simulink model "sampleModel140"  (R2021b)
settings: Solver=VariableStepAuto  StartTime=0.0  StopTime=10.0  RelTol=1e-3
undefined symbols (not defined in the file or in its folder): DiscIntNeverNeededParam, Newton, Raphson
libraries: simulink x11, slpidlib x1
settings Model: Creator=user  LastModifiedBy=user

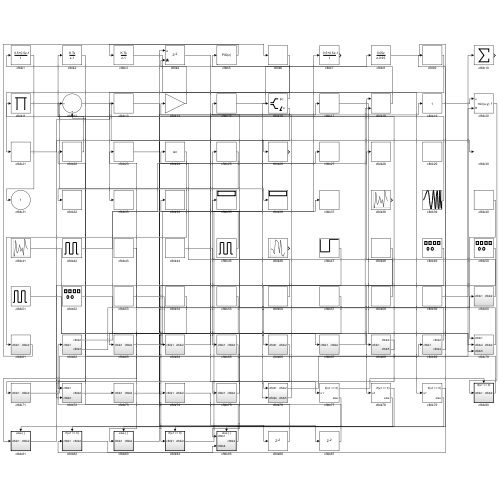
[thumbnail: Simulink's stored preview of the top-level diagram]
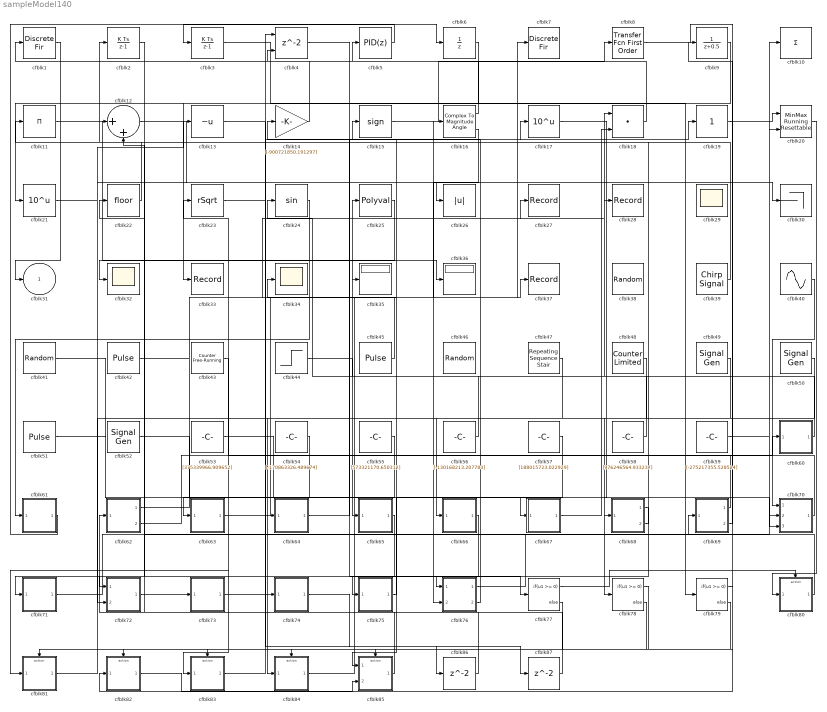
== system sampleModel140 ==
  cfblk1 : DiscreteFir  SampleTime=1
  cfblk10 : Sum  Inputs=+
  cfblk11 : Product  Inputs=*
  cfblk12 : Sum  Inputs=|++
  cfblk13 : UnaryMinus
  cfblk14 : Gain  Gain=[-900721850.191297]
  cfblk15 : Signum
  cfblk16 : ComplexToMagnitudeAngle
  cfblk17 : Math  Operator=10^u  SaturateOnIntegerOverflow=on
  cfblk18 : DotProduct  InputSameDT=on  OutDataTypeStr=Inherit: Inherit via internal rule
  cfblk19 : simulink/Math Operations/Slider Gain  gain=1  low=0  high=2
  cfblk2 : DiscreteIntegrator  ICPrevOutput=DiscIntNeverNeededParam  ICPrevScaledInput=DiscIntNeverNeededParam
  cfblk20 : simulink/Math Operations/MinMax Running Resettable  Function=min  vinit=0.0
  cfblk21 : Math  Operator=10^u  SaturateOnIntegerOverflow=on
  cfblk22 : Rounding
  cfblk23 : Sqrt  Operator=rSqrt  AlgorithmType=Newton-Raphson  SaturateOnIntegerOverflow=on
  cfblk24 : Trigonometry
  cfblk25 : Polyval  Coefs=[ +2.081618890e-019, -1.441693666e-014, +4.719686976e-010, -8.536869453e-006, +1.621573104e-001, -8.087801117e+001 ]
  cfblk26 : Abs
  cfblk27 : Record  FileSettingsInternal="{\"entries\":[{\"content\":{\"excelSettings\":{\"content\":{},\"type\":\"Streamout.ExcelSettings\"}},\"type\":\"Streamout.FileSettingStorage\",\"uuid\":\"f7dc172e-85bf-4364-b29a-430d7ad068c6\"}],\"packageUris\":[\"http://schema.mathworks.com/mf0/streamout_blocks/R2020a\"],\"version\":\"1.0\"}"  SignalsInternal="{\"entries\":[{\"content\":{\"signals\":[{\"content\":{\"blockPath\":[\"sampleModel140/cfblk27\"],\"channel\":[],\"dimensions\":[1],\"domain\":\"sampleModel140/cfblk27\",\"lineColor\":\"#fe330a\",\"plots\":[1],\"port\":1,\"sid\":[\"\"],\"signalID\":4999,\"signalName\":\"cfblk62:1\"},\"type\":\"RecordBlkView.Signal\",\"uuid\":\"44b31170-ca03-488e-82e6-39e71cb301d7\"}]},\"type\":\"RecordBlkView.InputSignals\",\"uuid\":\"1dfdc35e-76fa-4b09-975a-dfabfb6ba794\"}],\"packageUris\":[\"http://schema.mathworks.com/mf0/streamout_blocks/R2020a\"],\"version\":\"1.0\"}"  VisualizationBindings="{\"sparklinesplugin\":{\"info\":[{\"bindingParametersList\":[],\"subplotID\":1}]}}"
  cfblk28 : Record  FileSettingsInternal="{\"entries\":[{\"content\":{\"excelSettings\":{\"content\":{},\"type\":\"Streamout.ExcelSettings\"}},\"type\":\"Streamout.FileSettingStorage\",\"uuid\":\"2a60952b-dc02-4b89-ba4a-331db7f7e870\"}],\"packageUris\":[\"http://schema.mathworks.com/mf0/streamout_blocks/R2020a\"],\"version\":\"1.0\"}"  SignalsInternal="{\"entries\":[{\"content\":{\"signals\":[{\"content\":{\"blockPath\":[\"sampleModel140/cfblk28\"],\"channel\":[],\"dimensions\":[1],\"domain\":\"sampleModel140/cfblk28\",\"lineColor\":\"#22b573\",\"plots\":[1],\"port\":1,\"sid\":[\"\"],\"signalID\":5003,\"signalName\":\"cfblk73\"},\"type\":\"RecordBlkView.Signal\",\"uuid\":\"e06fc34c-2e52-42d5-b842-92c8cd7ea3f0\"}]},\"type\":\"RecordBlkView.InputSignals\",\"uuid\":\"c913dc81-a0a4-4d49-a666-7e3ebed671e0\"}],\"packageUris\":[\"http://schema.mathworks.com/mf0/streamout_blocks/R2020a\"],\"version\":\"1.0\"}"  VisualizationBindings="{\"sparklinesplugin\":{\"info\":[{\"bindingParametersList\":[],\"subplotID\":1}]}}"
  cfblk29 : Scope
      settings: Floating=on
  cfblk3 : DiscreteIntegrator  ICPrevOutput=DiscIntNeverNeededParam  ICPrevScaledInput=DiscIntNeverNeededParam
  cfblk30 : Terminator
  cfblk32 : Scope
  cfblk33 : Record  FileSettingsInternal="{\"entries\":[{\"content\":{\"excelSettings\":{\"content\":{},\"type\":\"Streamout.ExcelSettings\"}},\"type\":\"Streamout.FileSettingStorage\",\"uuid\":\"16210966-370f-487a-be88-b20549b0c51c\"}],\"packageUris\":[\"http://schema.mathworks.com/mf0/streamout_blocks/R2020a\"],\"version\":\"1.0\"}"  SignalsInternal="{\"entries\":[{\"content\":{\"signals\":[{\"content\":{\"blockPath\":[\"sampleModel140/cfblk33\"],\"channel\":[],\"dimensions\":[1],\"domain\":\"sampleModel140/cfblk33\",\"lineColor\":\"#0072bd\",\"plots\":[1],\"port\":1,\"sid\":[\"\"],\"signalID\":5007,\"signalName\":\"cfblk6\"},\"type\":\"RecordBlkView.Signal\",\"uuid\":\"1acb6f7d-3201-4389-8d54-da06513cf801\"}]},\"type\":\"RecordBlkView.InputSignals\",\"uuid\":\"1d47643f-2b85-4c86-9125-85e0580eef70\"}],\"packageUris\":[\"http://schema.mathworks.com/mf0/streamout_blocks/R2020a\"],\"version\":\"1.0\"}"  VisualizationBindings="{\"sparklinesplugin\":{\"info\":[{\"bindingParametersList\":[],\"subplotID\":1}]}}"
  cfblk34 : Scope
  cfblk35 : Display
  cfblk36 : Display
  cfblk37 : Record  FileSettingsInternal="{\"entries\":[{\"content\":{\"excelSettings\":{\"content\":{},\"type\":\"Streamout.ExcelSettings\"}},\"type\":\"Streamout.FileSettingStorage\",\"uuid\":\"14486def-ea98-4c8d-ac38-063aaeb98b28\"}],\"packageUris\":[\"http://schema.mathworks.com/mf0/streamout_blocks/R2020a\"],\"version\":\"1.0\"}"  SignalsInternal="{\"entries\":[{\"content\":{\"signals\":[{\"content\":{\"blockPath\":[\"sampleModel140/cfblk37\"],\"channel\":[],\"dimensions\":[1],\"domain\":\"sampleModel140/cfblk37\",\"lineColor\":\"#d95319\",\"plots\":[1],\"port\":1,\"sid\":[\"\"],\"signalID\":5011,\"signalName\":\"cfblk84\"},\"type\":\"RecordBlkView.Signal\",\"uuid\":\"8f6119ac-8ee8-4970-bbc5-a0b11d94bc15\"}]},\"type\":\"RecordBlkView.InputSignals\",\"uuid\":\"c6b40365-cea3-4913-9b63-00ff22d66e4e\"}],\"packageUris\":[\"http://schema.mathworks.com/mf0/streamout_blocks/R2020a\"],\"version\":\"1.0\"}"  VisualizationBindings="{\"sparklinesplugin\":{\"info\":[{\"bindingParametersList\":[],\"subplotID\":1}]}}"
  cfblk38 : UniformRandomNumber  Minimum=[-3035939554.229924]  Maximum=[4264926929.701888]  Seed=[60166904.000000]  SampleTime=0.1
  cfblk39 : simulink/Sources/Chirp Signal  f1=[917750893.399316]  T=[-110913934.255823]  f2=[-485528772.884929]
  cfblk4 : Delay  ShowEnablePort=on  SampleTime=1
      settings: InputPortMap=u0,e6
  cfblk40 : Sin  Amplitude=[-181022692.650693]  Bias=[660369983.554749]  SampleTime=0
  cfblk41 : UniformRandomNumber  Minimum=[-4870337137.228113]  Maximum=[9269629491.949644]  Seed=[65552154.000000]  SampleTime=0.1
  cfblk42 : DiscretePulseGenerator  PulseType=Time based  Amplitude=[-659661754.580511]  Period=[42044886.973960]  PulseWidth=5  PhaseDelay=[2.000000]
  cfblk43 : simulink/Sources/Counter Free-Running  NumBits=[5.000000]  tsamp=-1
  cfblk44 : Step  Time=[23.000000]  Before=[-869286196.761883]  After=[243619837.616728]  SampleTime=0
  cfblk45 : DiscretePulseGenerator  PulseType=Time based  Amplitude=[-997726001.498316]  Period=[30101274.943026]  PulseWidth=5  PhaseDelay=[1.000000]
  cfblk46 : RandomNumber  Mean=[-29909.071148]  Variance=[18577.204154]  Seed=[277614957.000000]  SampleTime=0.1
  cfblk47 : simulink/Sources/Repeating Sequence Stair  OutValues=[-714233188.830652, -476529493.049507]  tsamp=-1  OutMin=[]  OutMax=[]  OutDataTypeStr=double  OutputDataTypeScalingMode=double  OutDataType=fixdt(0,8)  ConRadixGroup=Best Precision: Vector-wise  OutScaling=2^-12
  cfblk48 : simulink/Sources/Counter Limited  uplimit=[364.000000]  tsamp=-1
  cfblk49 : SignalGenerator  WaveForm=square  Amplitude=[37695379.344834]  Units=rad/sec
  cfblk5 : slpidlib/PID Controller  Controller=PID  Form=Parallel  TimeDomain=Discrete-time  UseExternalTs=off  SampleTime=1  IntegratorMethod=Forward Euler  FilterMethod=Forward Euler  ControllerParametersSource=internal  P=1  I=1  D=0  UseFilter=on  N=100  TunerSelectOption=Transfer Function Based (PID Tuner App)  InitialConditionSource=internal  InitialConditionForIntegrator=0  InitialConditionForFilter=0  DifferentiatorICPrevScaledInput=0  ExternalReset=none  TrackingMode=off  Kt=1  LimitOutput=off  SatLimitsSource=internal  UpperSaturationLimit=inf  LowerSaturationLimit=-inf  LinearizeAsGain=off  AntiWindupMode=none  Kb=1  POutMin=[]  POutMax=[]  IOutMin=[]  IOutMax=[]  DOutMin=[]  DOutMax=[]  NOutMin=[]  NOutMax=[]  SumOutMin=[]  SumOutMax=[]  SaturationOutMin=[]  SaturationOutMax=[]  PParamMin=[]  PParamMax=[]  IParamMin=[]  IParamMax=[]  DParamMin=[]  DParamMax=[]  NParamMin=[]  NParamMax=[]  KbParamMin=[]  KbParamMax=[]  KtParamMin=[]  KtParamMax=[]  KbOutMin=[]  KbOutMax=[]  KtOutMin=[]  KtOutMax=[]  IntegratorOutMin=[]  IntegratorOutMax=[]  FilterOutMin=[]  FilterOutMax=[]  SumI1OutMin=[]  SumI1OutMax=[]  SumI2OutMin=[]  SumI2OutMax=[]  SumI3OutMin=[]  SumI3OutMax=[]  SumI4OutMin=[]  SumI4OutMax=[]  SumDOutMin=[]  SumDOutMax=[]  DifferentiatorOutMin=[]  DifferentiatorOutMax=[]  FilterDiffOutCoefMin=[]  FilterDiffOutCoefMax=[]  ReciprocalOutMin=[]  ReciprocalOutMax=[]  SumDenOutMin=[]  SumDenOutMax=[]  SumNumOutMin=[]  SumNumOutMax=[]  DivideOutMin=[]  DivideOutMax=[]  UdiffTsProdOutMin=[]  UdiffTsProdOutMax=[]  NTsProdOutMin=[]  NTsProdOutMax=[]  UintegralTsProdOutMin=[]  UintegralTsProdOutMax=[]  UngainTsProdOutMin=[]  UngainTsProdOutMax=[]  IntegratorContinuousStateAttributes=''  IntegratorStateMustResolveToSignalObject=off  IntegratorRTWStateStorageClass=Auto  FilterContinuousStateAttributes=''  FilterStateMustResolveToSignalObject=off  FilterRTWStateStorageClass=Auto  ParallelPVariant=InternalParameters  IdealPVariant=Disabled  IVariant=InternalParameters  DVariant=InternalParameters  IntegratorVariant=Discrete  SatVariant=Disabled  AWVariant=Passthrough  PCopyVariant=Disabled  TRVariant=Disabled  FdbkBlocksVariant=Forward  IdealPFdbkVariant=Disabled  SatFdbkVariant=Disabled  DerivativeFilterVariant=ForwardEulerFilter  NVariant=InternalParameters  NCopyVariant=Disabled  FilterICVariant=InternalICsFilter  IntegratorICVariant=InternalICs  ExternalResetVariant=Disabled  TRSumVariant=Passthrough  SumFdbkVariant=Disabled  SumVariant=Sum_PID  TsampFilterVariant=InternalTs  TsampNgainVariant=Passthrough  TsampIntegralVariant=Passthrough  ExternalSaturationOutDataTypeStr=Inherit: Same as second input
  cfblk50 : SignalGenerator  WaveForm=square  Amplitude=[-270396311.302956]
  cfblk51 : DiscretePulseGenerator  PulseType=Time based  Amplitude=[-700277655.752737]  Period=[70162605.232993]  PulseWidth=5  PhaseDelay=[7.000000]
  cfblk52 : SignalGenerator  WaveForm=sawtooth  Amplitude=[862125545.845058]
  cfblk53 : Constant  Value=[375339966.909652]  SampleTime=1
  cfblk54 : Constant  Value=[-170863326.489674]  SampleTime=1
  cfblk55 : Constant  Value=[573321170.650312]  SampleTime=1
  cfblk56 : Constant  Value=[-130168213.207783]  SampleTime=1
  cfblk57 : Constant  Value=[188015723.022929]  SampleTime=1
  cfblk58 : Constant  Value=[976246564.933237]  SampleTime=1
  cfblk59 : Constant  Value=[-275217355.528524]  SampleTime=1
  cfblk6 : UnitDelay  HasFrameUpgradeWarning=on
  cfblk60 : Subsystem
  cfblk61 : Subsystem
  cfblk62 : Subsystem
  cfblk63 : Subsystem
  cfblk64 : Subsystem
  cfblk65 : Subsystem
  cfblk66 : Subsystem
  cfblk67 : Subsystem
  cfblk68 : Subsystem
  cfblk69 : Subsystem
  cfblk7 : DiscreteFir  SampleTime=1
  cfblk70 : Subsystem
  cfblk71 : Subsystem
  cfblk72 : Subsystem
  cfblk73 : Subsystem
  cfblk74 : Subsystem
  cfblk75 : Subsystem
  cfblk76 : Subsystem
  cfblk77 : If  IfExpression=u1 >= 0  SampleTime=1
  cfblk78 : If  IfExpression=u1 >= 0  SampleTime=1
  cfblk79 : If  IfExpression=u1 >= 0  SampleTime=1
  cfblk8 : simulink/Discrete/Transfer Fcn First Order  PoleZ=0.95  ICPrevOutput=0.0  DoSatur=off
  cfblk80 : Subsystem  TreatAsAtomicUnit=on
  cfblk81 : Subsystem  TreatAsAtomicUnit=on
  cfblk82 : Subsystem  TreatAsAtomicUnit=on
  cfblk83 : Subsystem  TreatAsAtomicUnit=on
  cfblk84 : Subsystem  TreatAsAtomicUnit=on
  cfblk85 : Subsystem  TreatAsAtomicUnit=on
  cfblk86 : Delay  SampleTime=1
  cfblk87 : Delay  SampleTime=1
  cfblk9 : DiscreteTransferFcn  SampleTime=1
  cfblk31 : Outport
  wires:
  cfblk45/1 -> cfblk34/1
  cfblk62/1(cfblk2) -> cfblk27/1
  cfblk68/1(cfblk2) -> cfblk71/1(cfblk1)
  cfblk43/1 -> cfblk81/1(cfblk1)
  cfblk52/1 -> cfblk84/1(cfblk1)
  cfblk9/1 -> cfblk21/1
  cfblk6/1 -> cfblk33/1
  cfblk84/1(cfblk2) -> cfblk37/1
  cfblk8/1 -> cfblk82/1(cfblk1)
  cfblk60/1(cfblk2) -> cfblk24/1
  cfblk72/1(cfblk2) -> cfblk73/1(cfblk1)
  cfblk71/1(cfblk2) -> cfblk69/1(cfblk1)
  cfblk51/1 -> cfblk67/1(cfblk1)
  cfblk11/1 -> cfblk36/1
  cfblk83/1(cfblk2) -> cfblk17/1
  cfblk23/1 -> cfblk30/1
  cfblk25/1 -> cfblk32/1
  cfblk54/1 -> cfblk63/1(cfblk1)
  cfblk19/1 -> cfblk20/1
  cfblk63/1(cfblk2) -> cfblk7/1
  cfblk70/1(cfblk2) -> cfblk23/1
  cfblk22/1 -> cfblk2/1
  cfblk16/1 -> cfblk5/1
  cfblk15/1 -> cfblk8/1
  cfblk20/1 -> cfblk80/1(cfblk1)
  cfblk59/1 -> cfblk10/1
  cfblk56/1 -> cfblk25/1
  cfblk68/2(cfblk5) -> cfblk11/1
  cfblk12/1 -> cfblk74/1(cfblk1)
  cfblk69/1(cfblk2) -> cfblk15/1
  cfblk41/1 -> cfblk78/1
  cfblk24/1 -> cfblk61/1(cfblk1)
  cfblk49/1 -> cfblk68/1(cfblk1)
  cfblk44/1 -> cfblk65/1(cfblk1)
  cfblk76/1(cfblk2) -> cfblk20/2
  cfblk47/1 -> cfblk64/1(cfblk1)
  cfblk66/1(cfblk2) -> cfblk76/1(cfblk1)
  cfblk57/1 -> cfblk85/1(cfblk1)
  cfblk61/1(cfblk2) -> cfblk6/1
  cfblk40/1 -> cfblk70/1(cfblk1)
  cfblk76/2(cfblk5) -> cfblk14/1
  cfblk17/1 -> cfblk70/2(cfblk4)
  cfblk53/1 -> cfblk70/3(cfblk5)
  cfblk3/1 -> cfblk79/1
  cfblk69/2(cfblk4) -> cfblk9/1
  cfblk85/1(cfblk2) -> cfblk62/1(cfblk1)
  cfblk2/1 -> cfblk72/1(cfblk1)
  cfblk75/1(cfblk2) -> cfblk35/1
  cfblk80/1(cfblk2) -> cfblk22/1
  cfblk48/1 -> cfblk66/1(cfblk1)
  cfblk4/1 -> cfblk77/1
  cfblk21/1 -> cfblk26/1
  cfblk58/1 -> cfblk18/1
  cfblk18/1 -> cfblk4/2
  cfblk42/1 -> cfblk16/1
  cfblk55/1 -> cfblk83/1(cfblk1)
  cfblk62/2(cfblk3) -> cfblk60/1(cfblk1)
  cfblk14/1 -> cfblk1/1
  cfblk5/1 -> cfblk3/1
  cfblk50/1 -> cfblk72/2(cfblk3)
  cfblk1/1 -> cfblk31/1
  cfblk65/1(cfblk2) -> cfblk75/1(cfblk1)
  cfblk73/1(cfblk2) -> cfblk28/1
  cfblk39/1 -> cfblk12/1
  cfblk16/2 -> cfblk76/2(cfblk4)
  cfblk64/1(cfblk2) -> cfblk19/1
  cfblk81/1(cfblk2) -> cfblk13/1
  cfblk67/1(cfblk2) -> cfblk18/2
  cfblk82/1(cfblk2) -> cfblk85/2(cfblk4)
  cfblk77/1 -> cfblk80/Action
  cfblk77/2 -> cfblk81/Action
  cfblk78/1 -> cfblk82/Action
  cfblk78/2 -> cfblk83/Action
  cfblk79/1 -> cfblk84/Action
  cfblk79/2 -> cfblk85/Action
  cfblk13/1 -> cfblk86/1
  cfblk86/1 -> cfblk4/1
  cfblk74/1(cfblk2) -> cfblk87/1
  cfblk87/1 -> cfblk12/2

== system sampleModel140/cfblk60 ==
  cfblk1 : Inport
  cfblk3 : DiscreteFir  SampleTime=1
  cfblk2 : Outport
  wires:
  cfblk1/1 -> cfblk3/1
  cfblk3/1 -> cfblk2/1

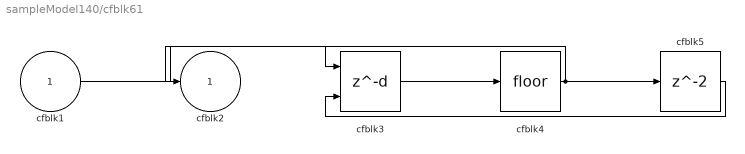
== system sampleModel140/cfblk61 ==
  cfblk1 : Inport
  cfblk3 : Delay  DelayLengthSource=Input port  SampleTime=1
      settings: InputPortMap=u0,p1
  cfblk4 : Rounding
  cfblk5 : Delay  SampleTime=1
  cfblk2 : Outport
  wires:
  cfblk1/1 -> cfblk3/1
  cfblk4/1 -> cfblk2/1, cfblk5/1
  cfblk3/1 -> cfblk4/1
  cfblk5/1 -> cfblk3/2

== system sampleModel140/cfblk62 ==
  cfblk1 : Inport
  cfblk2 : Outport
  cfblk3 : Outport  Port=2
  wires:
  cfblk1/1 -> cfblk2/1, cfblk3/1

== system sampleModel140/cfblk63 ==
  cfblk1 : Inport
  cfblk3 : Polyval  Coefs=[ +2.081618890e-019, -1.441693666e-014, +4.719686976e-010, -8.536869453e-006, +1.621573104e-001, -8.087801117e+001 ]
  cfblk2 : Outport
  wires:
  cfblk1/1 -> cfblk2/1, cfblk3/1

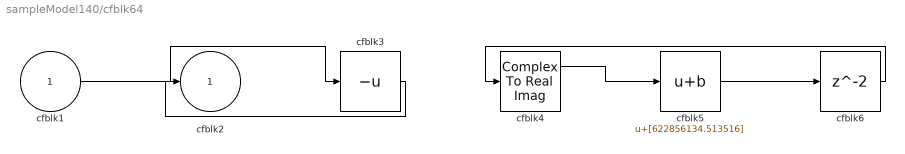
== system sampleModel140/cfblk64 ==
  cfblk1 : Inport
  cfblk3 : UnaryMinus
  cfblk4 : ComplexToRealImag
  cfblk5 : Bias  Bias=[622856134.513516]
  cfblk6 : Delay  SampleTime=1
  cfblk2 : Outport
  wires:
  cfblk1/1 -> cfblk3/1
  cfblk4/1 -> cfblk5/1
  cfblk3/1 -> cfblk2/1
  cfblk5/1 -> cfblk6/1
  cfblk6/1 -> cfblk4/1

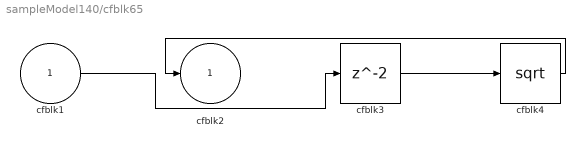
== system sampleModel140/cfblk65 ==
  cfblk1 : Inport
  cfblk3 : Delay  SampleTime=1
  cfblk4 : Sqrt  SaturateOnIntegerOverflow=on
  cfblk2 : Outport
  wires:
  cfblk3/1 -> cfblk4/1
  cfblk4/1 -> cfblk2/1
  cfblk1/1 -> cfblk3/1

== system sampleModel140/cfblk66 ==
  cfblk1 : Inport
  cfblk3 : Trigonometry
  cfblk4 : Constant  Value=[159650378.742997]  SampleTime=1
  cfblk2 : Outport
  wires:
  cfblk3/1 -> cfblk2/1
  cfblk4/1 -> cfblk3/1

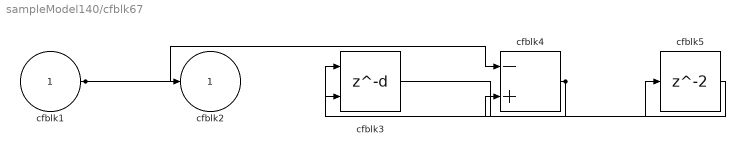
== system sampleModel140/cfblk67 ==
  cfblk1 : Inport
  cfblk3 : Delay  DelayLengthSource=Input port  SampleTime=1
      settings: InputPortMap=u0,p1
  cfblk4 : Sum  Inputs=-+
  cfblk5 : Delay  SampleTime=1
  cfblk2 : Outport
  wires:
  cfblk1/1 -> cfblk4/1, cfblk2/1
  cfblk4/1 -> cfblk3/1, cfblk3/2
  cfblk3/1 -> cfblk5/1
  cfblk5/1 -> cfblk4/2

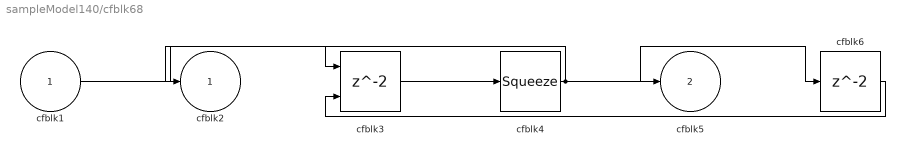
== system sampleModel140/cfblk68 ==
  cfblk1 : Inport
  cfblk3 : Delay  ShowEnablePort=on  SampleTime=1
      settings: InputPortMap=u0,e6
  cfblk4 : Squeeze
  cfblk6 : Delay  SampleTime=1
  cfblk2 : Outport
  cfblk5 : Outport  Port=2
  wires:
  cfblk1/1 -> cfblk3/1
  cfblk3/1 -> cfblk4/1
  cfblk4/1 -> cfblk5/1, cfblk2/1, cfblk6/1
  cfblk6/1 -> cfblk3/2

== system sampleModel140/cfblk69 ==
  cfblk1 : Inport
  cfblk3 : simulink/Discrete/Transfer Fcn Real Zero  ZeroZ=0.75  ICPrevInput=0.0  DoSatur=off
      settings: SourceProductBaseCode=SL
  cfblk2 : Outport
  cfblk4 : Outport  Port=2
  wires:
  cfblk1/1 -> cfblk4/1, cfblk3/1
  cfblk3/1 -> cfblk2/1

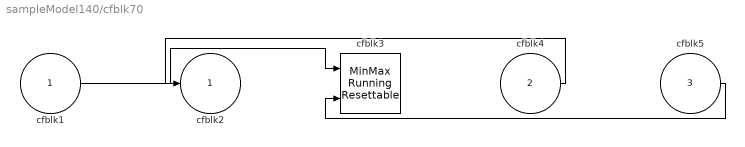
== system sampleModel140/cfblk70 ==
  cfblk1 : Inport
  cfblk4 : Inport  Port=2
  cfblk5 : Inport  Port=3
  cfblk3 : simulink/Math Operations/MinMax Running Resettable  Function=min  vinit=0.0
  cfblk2 : Outport
  wires:
  cfblk1/1 -> cfblk3/1
  cfblk5/1 -> cfblk3/2
  cfblk4/1 -> cfblk2/1

== system sampleModel140/cfblk71 ==
  cfblk1 : Inport
  cfblk3 : DiscreteZeroPole  Poles=[0 0.5]  Gain=1
  cfblk2 : Outport
  wires:
  cfblk1/1 -> cfblk2/1, cfblk3/1

== system sampleModel140/cfblk72 ==
  cfblk1 : Inport
  cfblk3 : Inport  Port=2
  cfblk2 : Outport
  wires:
  cfblk1/1 -> cfblk2/1

== system sampleModel140/cfblk73 ==
  cfblk1 : Inport
  cfblk3 : DiscreteStateSpace
  cfblk2 : Outport
  wires:
  cfblk3/1 -> cfblk2/1
  cfblk1/1 -> cfblk3/1

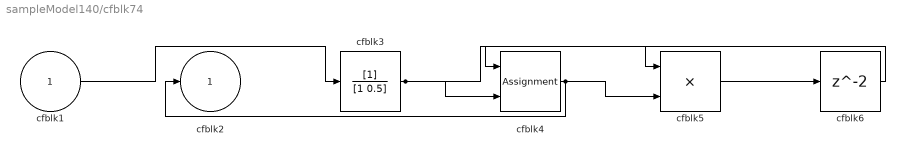
== system sampleModel140/cfblk74 ==
  cfblk1 : Inport
  cfblk3 : DiscreteFilter  SampleTime=1
  cfblk4 : Assignment  DiagnosticForDimensions=Warning  IndexOptions=Index vector (dialog)  Indices=1  OutputSizes=1
  cfblk5 : Product
  cfblk6 : Delay  SampleTime=1
  cfblk2 : Outport
  wires:
  cfblk3/1 -> cfblk4/2, cfblk5/1
  cfblk4/1 -> cfblk2/1, cfblk5/2
  cfblk1/1 -> cfblk3/1
  cfblk5/1 -> cfblk6/1
  cfblk6/1 -> cfblk4/1

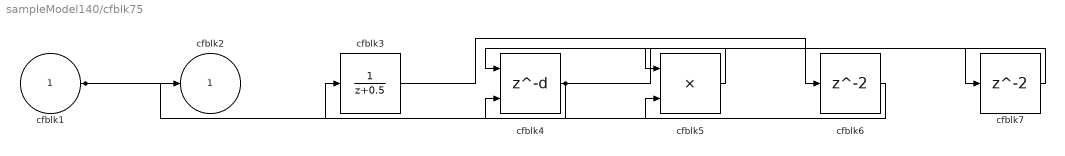
== system sampleModel140/cfblk75 ==
  cfblk1 : Inport
  cfblk3 : DiscreteTransferFcn  SampleTime=1
  cfblk4 : Delay  DelayLengthSource=Input port  SampleTime=1
      settings: InputPortMap=u0,p1
  cfblk5 : Product
  cfblk6 : Delay  SampleTime=1
  cfblk7 : Delay  SampleTime=1
  cfblk2 : Outport
  wires:
  cfblk5/1 -> cfblk4/1
  cfblk4/1 -> cfblk3/1, cfblk7/1
  cfblk1/1 -> cfblk2/1, cfblk5/2
  cfblk3/1 -> cfblk6/1
  cfblk6/1 -> cfblk4/2
  cfblk7/1 -> cfblk5/1

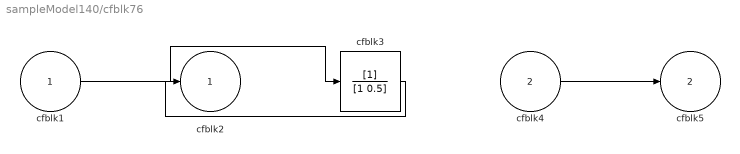
== system sampleModel140/cfblk76 ==
  cfblk1 : Inport
  cfblk4 : Inport  Port=2
  cfblk3 : DiscreteFilter  SampleTime=1
  cfblk2 : Outport
  cfblk5 : Outport  Port=2
  wires:
  cfblk1/1 -> cfblk3/1
  cfblk3/1 -> cfblk2/1
  cfblk4/1 -> cfblk5/1

== system sampleModel140/cfblk80 ==
  cfblk1 : Inport
  Action Port : ActionPort  ActionPortLabel=if(u1 >= 0)
  cfblk3 : simulink/Discrete/Difference  ICPrevInput=0.0  OutMin=[]  OutMax=[]  OutDataTypeStr=Inherit: Inherit via back propagation  OutDataType=fixdt(1, 16)  OutScaling=2^-10  DoSatur=off
  cfblk2 : Outport
  wires:
  cfblk3/1 -> cfblk2/1
  cfblk1/1 -> cfblk3/1

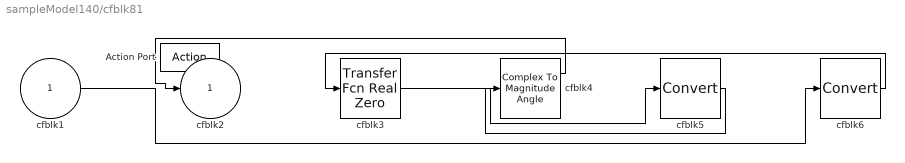
== system sampleModel140/cfblk81 ==
  cfblk1 : Inport
  Action Port : ActionPort  ActionPortLabel=else
  cfblk3 : simulink/Discrete/Transfer Fcn Real Zero  ZeroZ=0.75  ICPrevInput=0.0  DoSatur=off
      settings: SourceProductBaseCode=SL
  cfblk4 : ComplexToMagnitudeAngle
  cfblk5 : DataTypeConversion
  cfblk6 : DataTypeConversion
  cfblk2 : Outport
  wires:
  cfblk4/1 -> cfblk2/1
  cfblk3/1 -> cfblk5/1
  cfblk5/1 -> cfblk4/1
  cfblk1/1 -> cfblk6/1
  cfblk6/1 -> cfblk3/1

== system sampleModel140/cfblk82 ==
  cfblk1 : Inport
  Action Port : ActionPort  ActionPortLabel=if(u1 >= 0)
  cfblk3 : MinMax
  cfblk2 : Outport
  wires:
  cfblk1/1 -> cfblk3/1
  cfblk3/1 -> cfblk2/1

== system sampleModel140/cfblk83 ==
  cfblk1 : Inport
  Action Port : ActionPort  ActionPortLabel=else
  cfblk3 : UnaryMinus
  cfblk2 : Outport
  wires:
  cfblk1/1 -> cfblk3/1
  cfblk3/1 -> cfblk2/1

== system sampleModel140/cfblk84 ==
  cfblk1 : Inport
  Action Port : ActionPort  ActionPortLabel=if(u1 >= 0)
  cfblk3 : Constant  Value=[-871220624.482692]  SampleTime=1
  cfblk2 : Outport
  wires:
  cfblk3/1 -> cfblk2/1

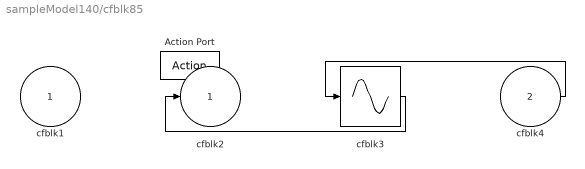
== system sampleModel140/cfblk85 ==
  cfblk1 : Inport
  cfblk4 : Inport  Port=2
  Action Port : ActionPort  ActionPortLabel=else
  cfblk3 : Sin  TimeSource=Use external signal  SampleTime=0
  cfblk2 : Outport
  wires:
  cfblk4/1 -> cfblk3/1
  cfblk3/1 -> cfblk2/1
